simulink model "sim_arm_pcont"  (R2023a)
settings: Solver=ode4  StartTime=0.0  StopTime=t(end)  FixedStep=0.001  RelTol=1e-3
values from neighbouring files (symbols this model uses):
  alpha1 = kP/wn^2    [ident_arm_2nd.m]    (also in ident_arm_lsm.m = p(1))
  delta1 = p(3)    [ident_arm_lsm.m]
  kP = 20    [arm_data.mat]
  mu1 = 2*zeta*wn*alpha1    [ident_arm_2nd.m]    (also in ident_arm_lsm.m = p(2))
undefined symbols (not defined in the file or in its folder): sgn
settings Model: Creator=kawata  LastModifiedBy=kawata
settings DataIOCC: ReturnWorkspaceOutputs=off
settings RTWCC: GPUComputeCapability=5.0

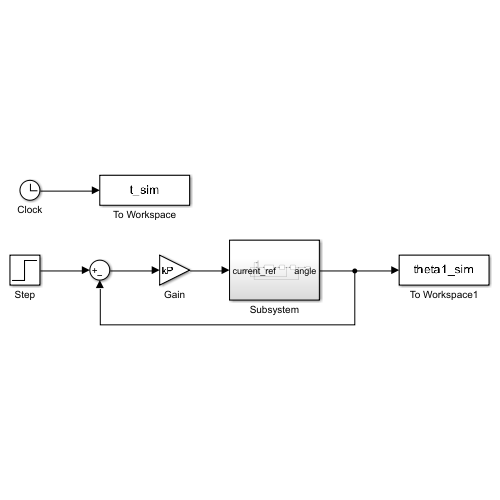
[thumbnail: Simulink's stored preview of the top-level diagram]
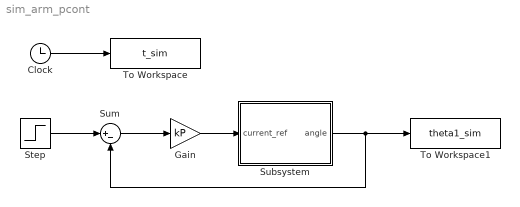
== system sim_arm_pcont ==
  Clock : Clock
  Gain : Gain  Gain=kP
  Step : Step  Time=0  After=r(end)  SampleTime=0
  Subsystem : Subsystem
  Sum : Sum  Inputs=|+-
  To Workspace : ToWorkspace  VariableName=t_sim  SampleTime=-1
  To Workspace1 : ToWorkspace  VariableName=theta1_sim  SampleTime=-1
  wires:
  Gain/1 -> Subsystem/1(current_ref)
  Sum/1 -> Gain/1
  Step/1 -> Sum/1
  Subsystem/1(angle) -> To Workspace1/1, Sum/2
  Clock/1 -> To Workspace/1

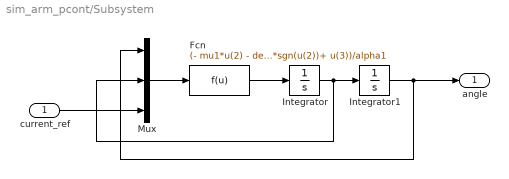
== system sim_arm_pcont/Subsystem ==
  current_ref : Inport
  Fcn : Fcn  Expr=(- mu1*u(2) - delta1*sgn(u(2))+ u(3))/alpha1
  Integrator : Integrator
  Integrator1 : Integrator
  Mux : Mux  Inputs=3
  angle : Outport
  wires:
  Integrator/1 -> Mux/2, Integrator1/1
  current_ref/1 -> Mux/3
  Fcn/1 -> Integrator/1
  Integrator1/1 -> Mux/1, angle/1
  Mux/1 -> Fcn/1
